simulink model "sampleModel1799"  (R2023a)
settings: Solver=VariableStepAuto  StartTime=0.0  StopTime=10.0  RelTol=1e-3
libraries: hdlsllib x6, simulink x3
settings Model: Creator=user1  LastModifiedBy=user1

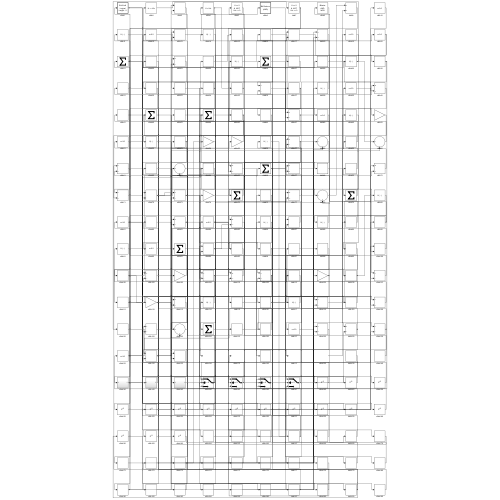
[thumbnail: Simulink's stored preview of the top-level diagram]
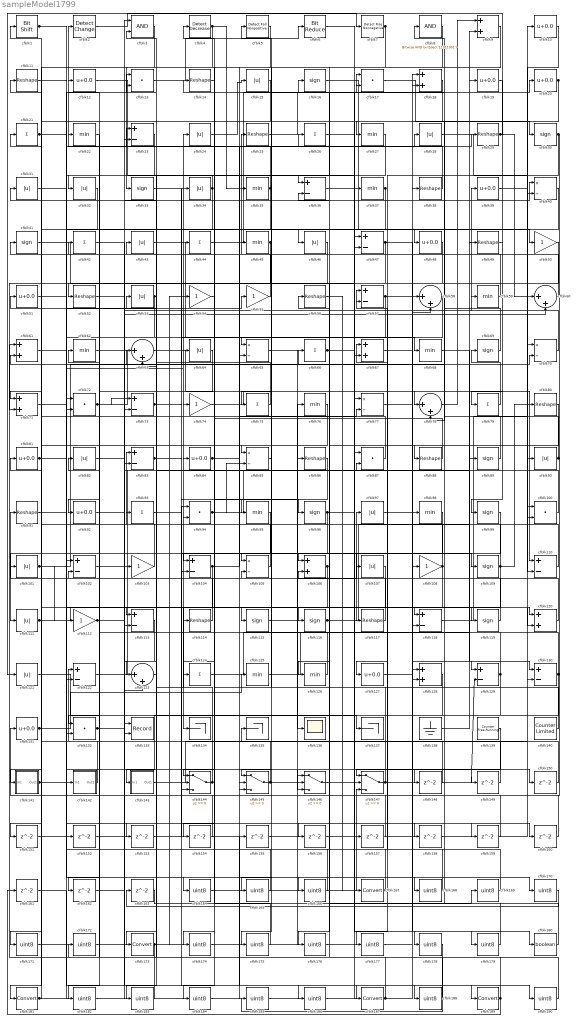
== system sampleModel1799 ==
  cfblk1 : hdlsllib/Logic and Bit Operations/Bit Shift  mode=Shift Left Logical  N=0
  cfblk{10,12,19..20,39,48,51,81,84,92,127,131} (12 alike) : Bias  Bias=0.0  SaturateOnIntegerOverflow=off
  cfblk{13,17,72,87,94,100,132} (7 alike) : DotProduct  OutDataTypeStr=Inherit: Inherit via internal rule
  cfblk{15,24,28,31..32,34,43,46,53,64,82,90,97,101,107,111,121} (17 alike) : Abs  SaturateOnIntegerOverflow=off
  cfblk{23,36,47,57,73,83,102,104,110,113,118,122,129..130} (14 alike) : Sum  Inputs=+-
  cfblk{50,54..55,74,103,108,112} (7 alike) : Gain
  cfblk{40,65,70,77,85,105} (6 alike) : Product  Inputs=*/  RndMeth=Zero  SaturateOnIntegerOverflow=on
  cfblk{9,18,61,67,71,106,120,128} (8 alike) : Sum
  cfblk{16,30,33,41,69,89,96,99,109,115..116,119} (12 alike) : Signum
  cfblk{11,14,25,29,38,49,52,56,80,86,88,91,114,117} (14 alike) : Reshape
  cfblk{58,60,63,78,123} (5 alike) : Sum  Inputs=|++
  cfblk{21,26,42,44,66,75,79,93,124} (9 alike) : Sum  Inputs=+
  cfblk{22,27,35,37,45,59,62,68,76,95,98,125..126} (13 alike) : MinMax
  cfblk133 : Record  FileSettingsInternal="{\"entries\":[{\"content\":{\"excelSettings\":{\"content\":{},\"type\":\"Streamout.ExcelSettings\"}},\"type\":\"Streamout.FileSettingStorage\",\"uuid\":\"\"}],\"packageUris\":[\"http:\\/\\/schema.mathworks.com\\/mf0\\/streamout_blocks\\/R2020a\"],\"version\":\"1.0\"}"  Layout=[1 1]  SignalsInternal="{\"entries\":[{\"content\":{\"signals\":[{\"content\":{\"blockPath\":[],\"dimensions\":[1],\"domain\":\"\",\"lineColor\":\"#a2142f\",\"plots\":[1],\"port\":1,\"signalID\":4129,\"signalName\":\"XY Graph:1\"},\"type\":\"RecordBlkView.Signal\",\"uuid\":\"\"},{\"content\":{\"blockPath\":[],\"dimensions\":[1],\"domain\":\"\",\"lineColor\":\"#139fff\",\"plots\":[1],\"port\":2,\"signalID\":4132,\"signalName\":\"XY Graph:2\"},\"type\":\"RecordBlkView.Signal\",\"uuid\":\"\"}]},\"type\":\"RecordBlkView.InputSignals\",\"uuid\":\"\"}],\"packageUris\":[\"http:\\/\\/schema.mathworks.com\\/mf0\\/streamout_blocks\\/R2020a\"],\"version\":\"1.0\"}"  VisualizationBindings="{\"xyplotplugin\":{\"info\":[{\"series\":[{\"bindingParametersList\":[{\"parameter\":\"X-Axis\",\"signalID\":4129,\"signalName\":\"XY Graph:1\"},{\"parameter\":\"Y-Axis\",\"signalID\":4132,\"signalName\":\"XY Graph:2\"}],\"seriesID\":53244}],\"subplotID\":1}]}}"  CompatibilityTag=XY  st=-1
  cfblk134 : Terminator
  cfblk135 : Terminator
  cfblk136 : Scope
  cfblk137 : Terminator
  cfblk138 : Ground
  cfblk139 : hdlsllib/Sources/Counter Free-Running  NumBits=16  tsamp=-1
  cfblk140 : hdlsllib/Sources/Counter Limited  uplimit=7  tsamp=-1
  cfblk141 : Subsystem
      settings: LibrarySourceBlock=|
      | hdlsllib/Ports &
      | Subsystems/Subsystem
  cfblk142 : Subsystem
      settings: LibrarySourceBlock=|
      | hdlsllib/Ports &
      | Subsystems/Subsystem
  cfblk143 : Subsystem
      settings: LibrarySourceBlock=|
      | hdlsllib/Ports &
      | Subsystems/Subsystem
  cfblk{144..147} (4 alike) : Switch  SaturateOnIntegerOverflow=off  InputSameDT=off
  cfblk{148..163} (16 alike) : Delay  SampleTime=1
  cfblk{164..166,168..172,174..179,182..186,188,190} (21 alike) : DataTypeConversion  OutDataTypeStr=uint8  SaturateOnIntegerOverflow=off  RndMeth=Floor
  cfblk{167,173,181,187,189} (5 alike) : DataTypeConversion  SaturateOnIntegerOverflow=off  RndMeth=Floor
  cfblk180 : DataTypeConversion  OutDataTypeStr=boolean  SaturateOnIntegerOverflow=off  RndMeth=Floor
  cfblk2 : simulink/Logic and Bit Operations/Detect Change  vinit=0  OutDataTypeStr=boolean
      settings: LibrarySourceBlock=|
      | hdlsllib/Logic and Bit
      | Operations/Detect
      | Change
  cfblk3 : Logic  AllPortsSameDT=off  OutDataTypeStr=boolean
  cfblk4 : simulink/Logic and Bit Operations/Detect Decrease  vinit=0.0  OutDataTypeStr=boolean
      settings: LibrarySourceBlock=|
      | hdlsllib/Logic and Bit
      | Operations/Detect
      | Decrease
  cfblk5 : hdlsllib/Logic and Bit Operations/Detect Fall Nonpositive  vinit=0  OutDataTypeStr=boolean
  cfblk6 : hdlsllib/Logic and Bit Operations/Bit Reduce  mode=AND
  cfblk7 : hdlsllib/Logic and Bit Operations/Detect Rise Nonnegative  vinit=0  OutDataTypeStr=boolean
  cfblk8 : simulink/Logic and Bit Operations/Bitwise Operator  logicop=AND  UseBitMask=on  BitMask=bin2dec('11011001')  BitMaskRealWorld=Stored Integer
      settings: LibrarySourceBlock=|
      | hdlsllib/Logic and Bit
      | Operations/Bitwise
      | Operator
  wires:
  cfblk144/1 -> cfblk24/1, cfblk31/1
  cfblk70/1 -> cfblk39/1
  cfblk121/1 -> cfblk137/1
  cfblk120/1 -> cfblk74/1
  cfblk44/1 -> cfblk17/1
  cfblk78/1 -> cfblk9/1
  cfblk114/1 -> cfblk91/1
  cfblk142/1(Out1) -> cfblk122/1
  cfblk146/1 -> cfblk77/1
  cfblk96/1 -> cfblk111/1, cfblk168/1
  cfblk43/1 -> cfblk65/1
  cfblk6/1 -> cfblk47/1
  cfblk74/1 -> cfblk78/1
  cfblk38/1 -> cfblk2/1
  cfblk16/1 -> cfblk48/1
  cfblk63/1 -> cfblk110/1
  cfblk105/1 -> cfblk81/1
  cfblk45/1 -> cfblk52/1, cfblk104/2
  cfblk83/1 -> cfblk145/3, cfblk183/1
  cfblk117/1 -> cfblk97/1
  cfblk60/1 -> cfblk25/1
  cfblk79/1 -> cfblk69/1
  cfblk116/1 -> cfblk49/1, cfblk120/1
  cfblk145/1 -> cfblk135/1, cfblk107/1
  cfblk107/1 -> cfblk134/1
  cfblk29/1 -> cfblk121/1, cfblk60/1
  cfblk54/1 -> cfblk104/1
  cfblk143/1(Out1) -> cfblk90/1
  cfblk131/1 -> cfblk125/1, cfblk156/1
  cfblk101/1 -> cfblk66/1, cfblk112/1
  cfblk32/1 -> cfblk101/1
  cfblk109/1 -> cfblk83/1, cfblk80/1, cfblk162/1
  cfblk122/1 -> cfblk9/2
  cfblk24/1 -> cfblk15/1
  cfblk28/1 -> cfblk110/2
  cfblk65/1 -> cfblk136/1
  cfblk129/1 -> cfblk67/1, cfblk154/1
  cfblk19/1 -> cfblk79/1
  cfblk68/1 -> cfblk130/1
  cfblk119/1 -> cfblk57/1
  cfblk3/1 -> cfblk33/1
  cfblk106/1 -> cfblk116/1, cfblk105/2
  cfblk85/1 -> cfblk145/1
  cfblk69/1 -> cfblk43/1
  cfblk52/1 -> cfblk83/2
  cfblk30/1 -> cfblk131/1, cfblk177/1
  cfblk34/1 -> cfblk32/1, cfblk144/3
  cfblk47/1 -> cfblk129/1, cfblk106/1
  cfblk58/1 -> cfblk105/1
  cfblk98/1 -> cfblk173/1
  cfblk112/1 -> cfblk123/2, cfblk188/1
  cfblk8/1 -> cfblk181/1
  cfblk27/1 -> cfblk123/1
  cfblk82/1 -> cfblk103/1
  cfblk108/1 -> cfblk45/1, cfblk127/1
  cfblk48/1 -> cfblk85/1
  cfblk42/1 -> cfblk189/1
  cfblk147/1 -> cfblk4/1, cfblk129/2
  cfblk12/1 -> cfblk47/2
  cfblk115/1 -> cfblk86/1
  cfblk113/1 -> cfblk133/2
  cfblk31/1 -> cfblk13/1
  cfblk104/1 -> cfblk29/1, cfblk141/1(In1)
  cfblk75/1 -> cfblk51/1
  cfblk125/1 -> cfblk37/1
  cfblk62/1 -> cfblk70/2
  cfblk73/1 -> cfblk96/1, cfblk109/1
  cfblk81/1 -> cfblk142/1(In1), cfblk146/3
  cfblk57/1 -> cfblk95/1, cfblk132/2, cfblk179/1
  cfblk71/1 -> cfblk28/1
  cfblk89/1 -> cfblk61/2
  cfblk39/1 -> cfblk100/2
  cfblk138/1 -> cfblk19/1
  cfblk132/1 -> cfblk40/1, cfblk59/1
  cfblk92/1 -> cfblk84/1
  cfblk66/1 -> cfblk20/1, cfblk126/1, cfblk149/1
  cfblk126/1 -> cfblk114/1
  cfblk17/1 -> cfblk30/1
  cfblk141/1(Out1) -> cfblk158/1, cfblk159/1
  cfblk1/1 -> cfblk50/1, cfblk119/1
  cfblk77/1 -> cfblk108/1
  cfblk103/1 -> cfblk62/1
  cfblk41/1 -> cfblk67/2
  cfblk40/1 -> cfblk46/1
  cfblk84/1 -> cfblk77/2, cfblk166/1, cfblk190/1
  cfblk100/1 -> cfblk53/1
  cfblk61/1 -> cfblk55/1
  cfblk86/1 -> cfblk144/1
  cfblk97/1 -> cfblk58/1
  cfblk56/1 -> cfblk167/1
  cfblk46/1 -> cfblk75/1
  cfblk118/1 -> cfblk10/1
  cfblk49/1 -> cfblk99/1
  cfblk64/1 -> cfblk92/1
  cfblk139/1 -> cfblk147/1
  cfblk9/1 -> cfblk65/2
  cfblk13/1 -> cfblk6/1
  cfblk111/1 -> cfblk115/1, cfblk64/1
  cfblk124/1 -> cfblk89/1
  cfblk88/1 -> cfblk44/1
  cfblk20/1 -> cfblk78/2, cfblk27/1
  cfblk36/1 -> cfblk118/1
  cfblk59/1 -> cfblk41/1
  cfblk123/1 -> cfblk63/1
  cfblk90/1 -> cfblk14/1, cfblk88/1
  cfblk130/1 -> cfblk82/1, cfblk143/1(In1)
  cfblk53/1 -> cfblk23/1, cfblk113/2
  cfblk110/1 -> cfblk16/1
  cfblk10/1 -> cfblk40/2
  cfblk23/1 -> cfblk72/2
  cfblk87/1 -> cfblk11/1
  cfblk25/1 -> cfblk17/2
  cfblk4/1 -> cfblk71/1, cfblk35/1
  cfblk50/1 -> cfblk71/2
  cfblk72/1 -> cfblk34/1, cfblk73/1, cfblk60/2
  cfblk33/1 -> cfblk68/1
  cfblk93/1 -> cfblk187/1
  cfblk2/1 -> cfblk7/1
  cfblk7/1 -> cfblk36/1, cfblk165/1
  cfblk35/1 -> cfblk113/1, cfblk3/2
  cfblk94/1 -> cfblk38/1, cfblk85/2
  cfblk140/1 -> cfblk5/1
  cfblk37/1 -> cfblk145/2, cfblk132/1
  cfblk95/1 -> cfblk122/2
  cfblk99/1 -> cfblk117/1
  cfblk21/1 -> cfblk120/2, cfblk153/1
  cfblk55/1 -> cfblk12/1
  cfblk5/1 -> cfblk124/1
  cfblk91/1 -> cfblk148/1
  cfblk148/1 -> cfblk72/1
  cfblk149/1 -> cfblk57/2
  cfblk51/1 -> cfblk150/1
  cfblk150/1 -> cfblk1/1
  cfblk15/1 -> cfblk151/1
  cfblk151/1 -> cfblk70/1
  cfblk152/1 -> cfblk23/2
  cfblk153/1 -> cfblk144/2
  cfblk154/1 -> cfblk3/1
  cfblk155/1 -> cfblk147/3
  cfblk156/1 -> cfblk100/1
  cfblk157/1 -> cfblk94/1
  cfblk158/1 -> cfblk130/2
  cfblk159/1 -> cfblk146/2
  cfblk127/1 -> cfblk160/1
  cfblk160/1 -> cfblk13/2
  cfblk162/1 -> cfblk73/2
  cfblk102/1 -> cfblk164/1
  cfblk164/1 -> cfblk157/1
  cfblk165/1 -> cfblk102/1
  cfblk166/1 -> cfblk102/2
  cfblk167/1 -> cfblk106/2, cfblk146/1
  cfblk168/1 -> cfblk56/1
  cfblk163/1 -> cfblk169/1
  cfblk169/1 -> cfblk87/2
  cfblk11/1 -> cfblk170/1
  cfblk170/1 -> cfblk163/1
  cfblk76/1 -> cfblk171/1
  cfblk171/1 -> cfblk87/1
  cfblk172/1 -> cfblk76/1
  cfblk173/1 -> cfblk172/1, cfblk54/1, cfblk58/2
  cfblk14/1 -> cfblk174/1
  cfblk174/1 -> cfblk98/1
  cfblk128/1 -> cfblk175/1
  cfblk175/1 -> cfblk94/2
  cfblk80/1 -> cfblk176/1
  cfblk176/1 -> cfblk128/1
  cfblk177/1 -> cfblk128/2
  cfblk26/1 -> cfblk178/1
  cfblk179/1 -> cfblk26/1
  cfblk67/1 -> cfblk180/1
  cfblk180/1 -> cfblk8/1
  cfblk181/1 -> cfblk152/1, cfblk21/1, cfblk133/1
  cfblk22/1 -> cfblk182/1
  cfblk182/1 -> cfblk155/1
  cfblk183/1 -> cfblk22/1
  cfblk18/1 -> cfblk184/1
  cfblk184/1 -> cfblk147/2
  cfblk178/1 -> cfblk185/1
  cfblk185/1 -> cfblk18/1
  cfblk161/1 -> cfblk186/1
  cfblk186/1 -> cfblk18/2
  cfblk187/1 -> cfblk118/2, cfblk63/2
  cfblk188/1 -> cfblk93/1
  cfblk189/1 -> cfblk161/1, cfblk36/2, cfblk61/1
  cfblk190/1 -> cfblk42/1

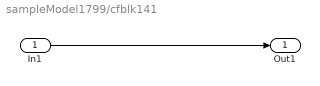
== system sampleModel1799/cfblk141 ==
  In1 : Inport
  Out1 : Outport
  wires:
  In1/1 -> Out1/1

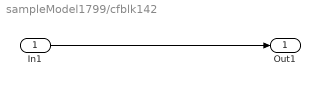
== system sampleModel1799/cfblk142 ==
  In1 : Inport
  Out1 : Outport
  wires:
  In1/1 -> Out1/1

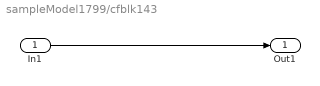
== system sampleModel1799/cfblk143 ==
  In1 : Inport
  Out1 : Outport
  wires:
  In1/1 -> Out1/1
